simulink model "MPC2019b"  (R2019b)
settings: Solver=FixedStepAuto  StartTime=0.0  StopTime=80  FixedStep=0.05  RelTol=1e-3
InitFcn:
  | startPose=[0,0,48]
StopFcn:
  | load('NewBaiYunPathDown6_13.mat')
  | n=1;
  | x0=0;
  | y0=0;
  | lng0 = BaiYunEmpty(2,1);
  | lat0 = BaiYunEmpty(1,1);
  | x1=[];
  | y1=[];
  | head=[];
  | nn = length(BaiYunEmpty(1,:));
  | while (n<nn)
  | lng2 = BaiYunEmpty(2,n);
  | lat2 = BaiYunEmpty(1,n);
  | head2 = BaiYunEmpty(3,n);
  | temp_x=(lng2-lng0)*111700*cos(lat2/180*pi);
  | temp_y=(lat2-lat0)*111700;
  | x1(n) = x0 + temp_x;
  | y1(n) = y0 + temp_y;
  | head(n)=head2;
  | n = n+1;
  | end
  | figure(1);
  | plot(x1,y1,'+r',out.v2(:,1),out.v2(:,2),'+k',out.v3(:,1),out.v3(:,2),'+b');
libraries: simulink x21, simulink_extras x4, drivingvehiclecontroller x2, vehdynlibsteering x2, autolibshared x2
(part 2 of 2)

== matlab function MPC2019b/Lateral_Control_Simulation-2/path_process1 ==
  data: curpoint input; speed_actual input; d output; v_tra output; steer_angle output; curvehhead input; curwheelangle input; curryawrate input; lateral_error output; heading_error output; H output; x output
function [d,v_tra,steer_angle,lateral_error,heading_error,H,x]  = fcn(curpoint,speed_actual,curvehhead,curwheelangle,curryawrate)
        %%s

R2D=57.2957805;
D2R=0.0174533;

dt = 0.05;

wheelbase_=2.9;
horizon_ = 10;
DIM_X = 4;
DIM_U = 1;
DIM_Y = 2;
u_lim = 30.0;
N = horizon_;

mass_fl = 600;
mass_fr = 600;
mass_rl = 600;
mass_rr = 600;


mass_front = mass_fl + mass_fr;
mass_rear = mass_rl + mass_rr;

mass_ = mass_front + mass_rear;
lf_ = wheelbase_ * (1.0 - mass_front / mass_);
lr_ = wheelbase_ * (1.0 - mass_rear / mass_);
iz_ = lf_ * lf_ * mass_front + lr_ * lr_ * mass_rear;
cf_= 155494.663;
cr_ = 155494.663;


%载入路径文件
Q = load('NewBaiYunPathDown6_13.mat');

dis_last = 100000;
abc=1;
abc_last = 1;
n=1;
x0=0;
y0=0;
lng0 = Q.BaiYunEmpty(2,1);
lat0 = Q.BaiYunEmpty(1,1);
temp_n = length(Q.BaiYunEmpty(1,:));

%%计算关键点
while (n<temp_n)    
lng2 = Q.BaiYunEmpty(2,n);
lat2 = Q.BaiYunEmpty(1,n);
temp_x=(lng2-lng0)*111700*cos(lat2/180*pi);
temp_y=(lat2-lat0)*111700;    
x1 = x0 + temp_x;
y1 = y0 + temp_y;
x2=curpoint(1);
y2=curpoint(2);
    dis=sqrt((x1-x2)^2+(y1-y2)^2);
    if(dis<dis_last)
        abc=n;
        dis_last = dis;
    else
        abc=abc_last;
    end
abc_last = abc;
n = n+1;
end
keypointlist = abc;%得到关键点id
%%计算关键点和关键点前一点的xy
key_x=(Q.BaiYunEmpty(2,keypointlist)-lng0)*111700*cos(Q.BaiYunEmpty(1,keypointlist)/180*pi);
key_y=(Q.BaiYunEmpty(1,keypointlist)-lat0)*111700; 
key_theta=Q.BaiYunEmpty(3,keypointlist);
key_x1=(Q.BaiYunEmpty(2,keypointlist+1)-lng0)*111700*cos(Q.BaiYunEmpty(1,keypointlist+1)/180*pi);
key_y1=(Q.BaiYunEmpty(1,keypointlist+1)-lat0)*111700; 
key_delta_x = key_x - curpoint(1);
key_delta_y = key_y - curpoint(2);
key_delta_x1 = key_x1 - curpoint(1);
key_delta_y1 = key_y1 - curpoint(2);
%%计算横向偏差
dis1 = sqrt((key_delta_x1)^2+(key_delta_y1)^2);
dis2 = sqrt((key_x1-key_x)^2+(key_y1-key_y)^2);
area = 1/4*sqrt((dis_last+dis1+dis2)*(dis_last+dis1-dis2)*(dis_last+dis2-dis1)*(dis1+dis2-dis_last));
if(dis2>=0.01)
    d=2.0*area/dis2;
else
    d=dis_last;
end      

if(key_delta_x>-0.0001&&key_delta_x<0.0001)
    if(key_delta_y>0)
        key_point_direction=0;
    else
        key_point_direction=180;
    end    
else    
   key_point_direction = atan(key_delta_y / key_delta_x) / pi*180;
    if (key_delta_x > 0) 
        key_point_direction = 90 - key_point_direction;
    else
        key_point_direction = 270 - key_point_direction;
    end
end

%%计算关键点附近曲率
n=1;
Larc=0;
while(n<=5)
Larc_add = getDistance(Q.BaiYunEmpty(1,keypointlist),Q.BaiYunEmpty(2,keypointlist),Q.BaiYunEmpty(1,keypointlist+n),Q.BaiYunEmpty(2,keypointlist+n));    
Larc = Larc+Larc_add;
n=n+1;
end
delta_head = Q.BaiYunEmpty(3,keypointlist+5)-Q.BaiYunEmpty(3,keypointlist);
kappa = delta_head*D2R/Larc;
kappa = max(min(kappa,0.1),-0.1);
curvature_=kappa;
v_tra = Q.BaiYunEmpty(4,keypointlist);
%%%%%%%%%%%%%%%%%%%

%%apollo横向偏差计算
dx_apo = curpoint(1) - key_x;
dy_apo = curpoint(2) - key_y;
cos_target_heading = cos(key_theta*D2R);
sin_target_heading = sin(key_theta*D2R);
%%%%状态量%%%%%%
lateral_error = cos_target_heading * dy_apo - sin_target_heading * dx_apo;
heading_error = key_theta - curvehhead;
lateral_error_dot = speed_actual*sin(heading_error);
heading_error_rate = kappa*speed_actual - curryawrate;
%%%%%%%%%%%%%%%%%
x0 = zeros(4,1);
x0(1, 1) = lateral_error;
x0(2, 1) = lateral_error_dot;
x0(3, 1) = heading_error;
x0(4, 1) = heading_error_rate;

Aex = zeros(DIM_X * N, DIM_X);
Bex = zeros(DIM_X * N, DIM_U * N);
Wex = zeros(DIM_X * N, 1);
Cex = zeros(DIM_Y * N, DIM_X * N);
Qex = zeros(DIM_Y * N, DIM_Y * N);
Rex = zeros(DIM_U * N, DIM_U * N);
Urefex = zeros(DIM_U * N, 1);

% Aex = cell(N,1);
% Bex = cell(N,N);
% Wex = cell(N,1);
% Cex = cell(N,N);
% Qex = cell(N,N);
% Rex = cell(N,N);
% Urefex = cell(N,1);


Q = zeros(DIM_Y, DIM_Y);
R = zeros(DIM_U, DIM_U);
Q(1, 1) = 0.01;
Q(2, 2) = 0.01;
R(1, 1) = 1;
% Q_adaptive = zeros(DIM_Y, DIM_Y);
% R_adaptive = zeros(DIM_U, DIM_U);
Q_adaptive = Q;
R_adaptive = R;

vel=max(1,speed_actual);

Ad = zeros(DIM_X, DIM_X);
Ad(1, 2) = 1.0;
Ad(2, 2) = -(cf_ + cr_) / (mass_ * vel);
Ad(2, 3) = (cf_ + cr_) / mass_;
Ad(2, 4) = (lr_ * cr_ - lf_ * cf_) / (mass_ * vel);
Ad(3, 4) = 1.0;
Ad(4, 2) = (lr_ * cr_ - lf_ * cf_) / (iz_ * vel);
Ad(4, 3) = (lf_ * cf_ - lr_ * cr_) / iz_;
Ad(4, 4) = -(lf_ * lf_ * cf_ + lr_ * lr_ * cr_) / (iz_ * vel);

I=eye(DIM_X,DIM_X);
Ad_inverse = inv(I - dt * 0.5 * Ad);
Ad = (I - dt * 0.5 * Ad)\(I + dt * 0.5 * Ad);

Bd = zeros(DIM_X,DIM_U);
Bd(1, 1) = 0.0;
Bd(2, 1) = cf_ / mass_;
Bd(3, 1) = 0.0;
Bd(4, 1) = lf_ * cf_ / iz_;

Wd = zeros(DIM_X, 1);
Wd(1, 1) = 0.0;
Wd(2, 1) = (lr_ * cr_ - lf_ * cf_) / (mass_ * vel) - vel;
Wd(3, 1) = 0.0;
Wd(4, 1) = -(lf_ * lf_ * cf_ + lr_ * lr_ * cr_) / (iz_ * vel);

Cd = zeros(DIM_Y, DIM_X);
Cd(1, 1) = 1.0;
Cd(2, 3) = 1.0;

%curvature_ = 0.0;

Bd = (Ad_inverse * dt) * Bd;
Wd = (Ad_inverse * dt * curvature_ * vel) * Wd;

%  for j=1:1:N
%     Aex{j,1}=Ad^j;
%     if(j==1)
%         Wex{j,1} = Wd;
%     else
%         Wex{j,1}=Ad^(j-1)*Wd+Wex{j-1,1};
%     end
%     for k=1:1:N
%        if k<=j
%             Bex{j,k}=(Ad^(j-k))*Bd;
%        else
%             Bex{j,k}=zeros(Nx,Nu);
%        end
%     end
%     Cex(idx_y_i+1:idx_y_i+DIM_Y, idx_x_i+1:idx_x_i+DIM_X) = Cd;
%     Qex(idx_y_i+1:idx_y_i+DIM_Y, idx_y_i+1:idx_y_i+DIM_Y) = Q_adaptive;
%     Rex(idx_u_i+1:idx_u_i+DIM_U, idx_u_i+1:idx_u_i+DIM_U) = R_adaptive;
% end



for i=0:1:N-1

    %update mpc matrix
    idx_x_i = i * DIM_X;
    idx_x_i_prev = (i - 1) * DIM_X;
    idx_u_i = i * DIM_U;
    idx_y_i = i * DIM_Y;
    if (i == 0)  
      Aex(1:DIM_X,1:DIM_X) = Ad;
      Bex(1:DIM_X,1:DIM_U) = Bd;
      Wex(1:DIM_X,1:1) = Wd;
    else
        Aex(idx_x_i+1:idx_x_i+DIM_X,1:DIM_X) = Ad * Aex(idx_x_i_prev+1:idx_x_i_prev+DIM_X,1:DIM_X);
      for j = 0:1:i-1
        idx_u_j = j * DIM_U;
        Bex(idx_x_i+1:idx_x_i+DIM_X, idx_u_j+1:idx_u_j+DIM_U) = Ad * Bex(idx_x_i_prev+1:idx_x_i_prev+DIM_X, idx_u_j+1:idx_u_j+DIM_U);
      end
      Wex(idx_x_i+1:idx_x_i+DIM_X, 1:1) = Ad * Wex(idx_x_i_prev+1:idx_x_i_prev+DIM_X, 1:1) + Wd;
      
    end
    Bex(idx_x_i+1:idx_x_i+DIM_X, idx_u_i+1:idx_u_i+DIM_U) = Bd;
    Cex(idx_y_i+1:idx_y_i+DIM_Y, idx_x_i+1:idx_x_i+DIM_X) = Cd;
    Qex(idx_y_i+1:idx_y_i+DIM_Y, idx_y_i+1:idx_y_i+DIM_Y) = Q_adaptive;
    Rex(idx_u_i+1:idx_u_i+DIM_U, idx_u_i+1:idx_u_i+DIM_U) = R_adaptive;

kv = lr_ * mass_ / 2 / cf_ / wheelbase_ - lf_ * mass_ / 2 / cr_ / wheelbase_;
Uref = wheelbase_ * kappa + kv * vel * vel * kappa;
Urefex(i*DIM_U+1 : i*DIM_U+DIM_U, 1:1) = Uref;

end



%%%%%%%%%%%%%%%%%optimization%%%%%%%%%%%%%%%%%%%%%%
CB = Cex * Bex;
QCB = Qex * CB;
% H = zeros(DIM_U * N, DIM_U * N);
H = CB' * QCB + Rex;
f = (Cex * (Aex * x0 + Wex))' * QCB - Urefex'* Rex;

%%constraint matrix : lb < U < ub, lbA < A*U < ubA 
A = zeros(DIM_U * N, DIM_U * N);
lbA = zeros(DIM_U * N, 1);
ubA = zeros(DIM_U * N, 1);
lb = linspace(-u_lim*D2R, -u_lim*D2R, DIM_U * N);
ub = linspace(u_lim*D2R, u_lim*D2R, DIM_U * N);
g=f';
%%%%%%%%%%%%%%%%%%%%%%%%%solver%%%%%%%%%%%%%%%%%%%%%%%%%%%%%%%%%%%%%%%%%%%
kNumOfMatrixElements = size(H,1) * size(H,2);
h_matrix = zeros(1,kNumOfMatrixElements);
kNumOfOffsetRows = size(g,1);
g_matrix = zeros(1,kNumOfOffsetRows);
lower_bound = zeros(1,kNumOfOffsetRows);
upper_bound = zeros(1,kNumOfOffsetRows);
Aconstraint = eye(kNumOfOffsetRows, kNumOfOffsetRows);
a_constraint_matirx = zeros(1,kNumOfMatrixElements);

index = 1;

for  r = 0:1:size(H,1)-1
    g_matrix(1,r+1) = g(r+1, 1);
for c = 0:1:size(H,2)-1
  h_matrix(index) = H(r+1, c+1);
  a_constraint_matirx(1,index) = Aconstraint(r+1, c+1);
  index = index + 1;
end
end

%   for i = 0:1:kNumOfOffsetRows-1
%     lower_bound(1,i+1) = lb(i+1);
%     upper_bound(1,i+1) = ub(i+1);
%   end


options = optimoptions(@quadprog,'Algorithm','active-set');
%%options = optimset('active-set');
x_start=ones(N,1);
x = quadprog(H,g,Aconstraint,ub,[],[],lb,ub,x_start,options);



u_sat = max(min(x(1), u_lim*D2R), -u_lim*D2R);
steer_cmd = u_sat*R2D;
steer_angle = steer_cmd;%steer_angle_feedback+steer_angle_feedforwardterm;



end

function result_angle = getAngleByTwoGps(lat1, lng1, lat2, lng2)
R2D=57.2957805;
D2R=0.0174533;
dx = (lng2 - lng1) * 111700 *cos(lat1*D2R);
dy = (lat2 - lat1) * 111700;

result_angle = atan2(dx,dy)*R2D;%%计算与y轴正方向的夹角(-180~180)
if(result_angle <0)
    result_angle = 360+result_angle;
end
end

function Dis = getDistance(lat1,lng1,lat2,lng2)

    x=abs(lng1-lng2)*111700*cos(lat1/180*3.141592653589793);
    y=abs(lat1-lat2)*111700;

    Dis=sqrt(x*x+y*y);
end
